simulink model "testRam"  (R2015a)
settings: Solver=ode45  StartTime=0.0  StopTime=10.0  RelTol=1e-3
InitFcn:
  | %% DSPBuilder Start
  | alt_dspbuilder_update_model(bdroot)
  | %% DSPBuilder End
libraries: allblocks_alteradspbuilder2 x35
settings Model: Creator=ASUS  LastModifiedBy=ASUS

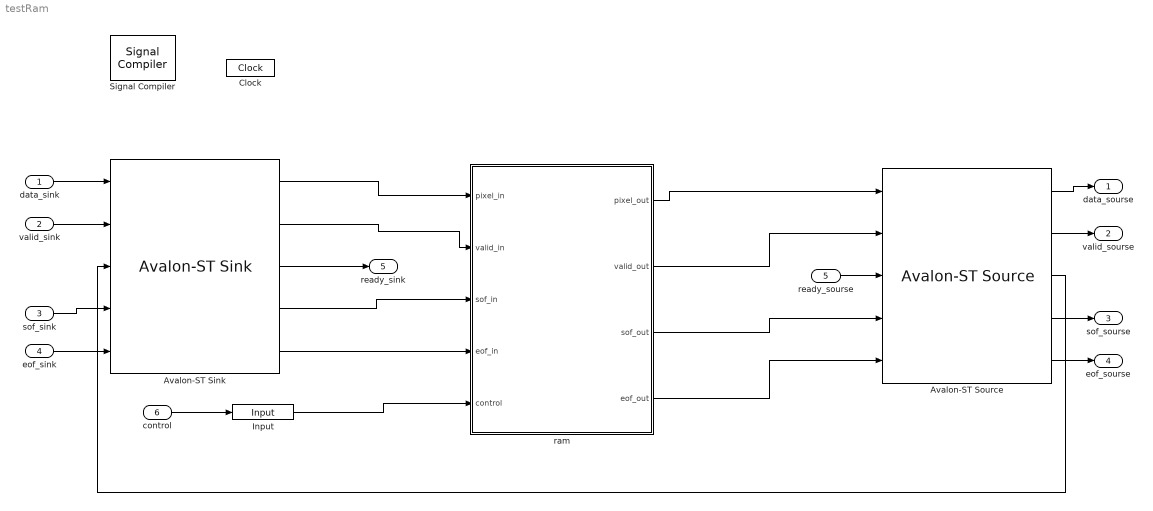
== system testRam ==
  data_sink : Inport
  valid_sink : Inport  Port=2
  sof_sink : Inport  Port=3
  eof_sink : Inport  Port=4
  ready_sourse : Inport  Port=5
  control : Inport  Port=6
  Avalon-ST Sink : allblocks_alteradspbuilder2/Avalon-ST Sink  iofile=C:\Users\ASUS\Desktop\sift_fpga\Octave_2\tb_testRam\testRam_Avalon-ST+Sink_data.salt,C:\Users\ASUS\Desktop\sift_fpga\Octave_2\tb_testRam\testRam_Avalon-ST+Sink_valid.salt,C:\Users\ASUS\Desktop\sift_fpga\Octave_2\tb_testRam\testRam_Avalon-ST+Sink_ready.capture,C:\Users\ASUS\Desktop\sift_fpga\Octave_2\tb_testRam\testRam_Avalon-ST+Sink_startofpacket.salt,C:\Users\ASUS\Desktop\sift_fpga\Octave_2\tb_testRam\testRam_Avalon-ST+Sink_endofpacket.salt,  SpecifyClock=off  BusType=Unsigned Integer  bwl=24  bwr=0  symbolWidth=8  symbolsPerBeat=3  numOfChannels=0  numOfErrorDescriptors=0  endOfPacket=on  startOfPacket=on  empty=off  readyLatency=1  externalType=Inferred  PORTTYPE=Output
  Avalon-ST Source : allblocks_alteradspbuilder2/Avalon-ST Source  iofile=C:\Users\ASUS\Desktop\sift_fpga\Octave_2\tb_testRam\testRam_Avalon-ST+Source_data.capture,C:\Users\ASUS\Desktop\sift_fpga\Octave_2\tb_testRam\testRam_Avalon-ST+Source_valid.capture,C:\Users\ASUS\Desktop\sift_fpga\Octave_2\tb_testRam\testRam_Avalon-ST+Source_ready.salt,C:\Users\ASUS\Desktop\sift_fpga\Octave_2\tb_testRam\testRam_Avalon-ST+Source_startofpacket.capture,C:\Users\ASUS\Desktop\sift_fpga\Octave_2\tb_testRam\testRam_Avalon-ST+Source_endofpacket.capture,  SpecifyClock=off  BusType=Unsigned Integer  bwl=24  bwr=0  symbolWidth=8  symbolsPerBeat=3  numOfChannels=0  numOfErrorDescriptors=0  endOfPacket=on  startOfPacket=on  empty=off  readyLatency=1  externalType=Inferred  PORTTYPE=Input
  Clock : allblocks_alteradspbuilder2/Clock  ClockPeriod=10/1.5  ClockPeriodUnit=ns  SampleTime=1  ResetLatency=0  ResetRegisterCascadeDepth=0  SimulationStartCycle=5  PhaseOffset=0  Reset=aclr  ResetType=Active Low  Export=off
  Input : allblocks_alteradspbuilder2/Input  iofile=C:\Users\ASUS\Desktop\sift_fpga\Octave_2\tb_testRam\testRam_Input.salt  BusType=Unsigned Integer  bwl=18  bwr=0  SpecifyClock=off  PORTTYPE=Input  externalType=Inferred  allowFloatingPointOverride=on  logOutputs=off
  Signal Compiler : allblocks_alteradspbuilder2/Signal Compiler  DeviceFamily=Cyclone IV GX  DeviceName=AUTO  DisableEarlyHDLGeneration=off  EnableSignalTap=off  SignalTapDepth=128  UseBoardBlock=off  StpUseDefaultClock=on  StpClock=Clock  ExportDir=C:\altera\16.0\quartus\dsp_builder  MAX10_ProgrammingMode=Internal Flash (SDM) Single Boot
  ram : Subsystem
  data_sourse : Outport
  valid_sourse : Outport  Port=2
  sof_sourse : Outport  Port=3
  eof_sourse : Outport  Port=4
  ready_sink : Outport  Port=5
  wires:
  ram/1(pixel_out) -> Avalon-ST Source/1
  Avalon-ST Sink/1 -> ram/1(pixel_in)
  Avalon-ST Sink/2 -> ram/2(valid_in)
  ram/2(valid_out) -> Avalon-ST Source/2
  ram/3(sof_out) -> Avalon-ST Source/4
  ram/4(eof_out) -> Avalon-ST Source/5
  Avalon-ST Sink/5 -> ram/4(eof_in)
  Avalon-ST Sink/4 -> ram/3(sof_in)
  Avalon-ST Source/3 -> Avalon-ST Sink/3
  Avalon-ST Source/1 -> data_sourse/1
  Avalon-ST Source/2 -> valid_sourse/1
  Avalon-ST Source/4 -> sof_sourse/1
  Avalon-ST Source/5 -> eof_sourse/1
  data_sink/1 -> Avalon-ST Sink/1
  valid_sink/1 -> Avalon-ST Sink/2
  sof_sink/1 -> Avalon-ST Sink/4
  eof_sink/1 -> Avalon-ST Sink/5
  ready_sourse/1 -> Avalon-ST Source/3
  Avalon-ST Sink/3 -> ready_sink/1
  control/1 -> Input/1
  Input/1 -> ram/5(control)

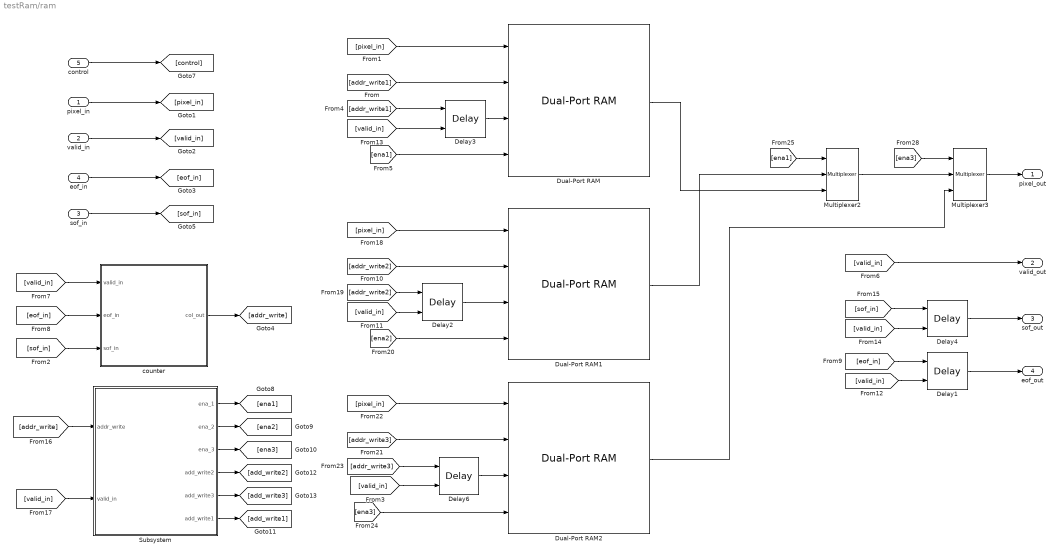
== system testRam/ram ==
  pixel_in : Inport
  valid_in : Inport  Port=2
  sof_in : Inport  Port=3
  eof_in : Inport  Port=4
  control : Inport  Port=5
  Delay1 : allblocks_alteradspbuilder2/Delay  pipeline=5  pipeline_display=5  ClockPhase=1  use_ena=on  use_sclr=off  allowFloatingPointOverride=on  logOutputs=off  logFile=C:\Users\ASUS\Desktop\sift_fpga\Octave_2\tb_testRam\testRam_ram_Delay1.fixedpointlog  use_init=off  reset_value=1
  Delay2 : allblocks_alteradspbuilder2/Delay  pipeline=1  pipeline_display=1  ClockPhase=1  use_ena=on  use_sclr=off  allowFloatingPointOverride=on  logOutputs=off  logFile=C:\Users\ASUS\Desktop\sift_fpga\Octave_2\tb_testRam\testRam_ram_Delay2.fixedpointlog  use_init=off  reset_value=1
  Delay3 : allblocks_alteradspbuilder2/Delay  pipeline=1  pipeline_display=1  ClockPhase=1  use_ena=on  use_sclr=off  allowFloatingPointOverride=on  logOutputs=off  logFile=C:\Users\ASUS\Desktop\sift_fpga\Octave_2\tb_testRam\testRam_ram_Delay3.fixedpointlog  use_init=off  reset_value=1
  Delay4 : allblocks_alteradspbuilder2/Delay  pipeline=5  pipeline_display=5  ClockPhase=1  use_ena=on  use_sclr=off  allowFloatingPointOverride=on  logOutputs=off  logFile=C:\Users\ASUS\Desktop\sift_fpga\Octave_2\tb_testRam\testRam_ram_Delay4.fixedpointlog  use_init=off  reset_value=1
  Delay6 : allblocks_alteradspbuilder2/Delay  pipeline=1  pipeline_display=1  ClockPhase=1  use_ena=on  use_sclr=off  allowFloatingPointOverride=on  logOutputs=off  logFile=C:\Users\ASUS\Desktop\sift_fpga\Octave_2\tb_testRam\testRam_ram_Delay6.fixedpointlog  use_init=off  reset_value=1
  Dual-Port RAM : allblocks_alteradspbuilder2/Dual-Port RAM  numwords=10000  BusType=Unsigned Integer  bwl=24  bwr=0  memory_type=M10K  ram_type=DualRAM  dont_care=off  initialization=Blank  init_file=input.hex  init_array=[0:1:15]  register_outputs=on  use_ena=off  ClockPhase=1  allowFloatingPointOverride=on  logOutputs=off  logFile=C:\Users\ASUS\Desktop\sift_fpga\Octave_2\tb_testRam\testRam_ram_Dual-Port+RAM.fixedpointlog  pipeline_display=2
  Dual-Port RAM1 : allblocks_alteradspbuilder2/Dual-Port RAM  numwords=10000  BusType=Unsigned Integer  bwl=24  bwr=0  memory_type=M10K  ram_type=DualRAM  dont_care=off  initialization=Blank  init_file=input.hex  init_array=[0:1:15]  register_outputs=on  use_ena=off  ClockPhase=1  allowFloatingPointOverride=on  logOutputs=off  logFile=C:\Users\ASUS\Desktop\sift_fpga\Octave_2\tb_testRam\testRam_ram_Dual-Port+RAM1.fixedpointlog  pipeline_display=2
  Dual-Port RAM2 : allblocks_alteradspbuilder2/Dual-Port RAM  numwords=10000  BusType=Unsigned Integer  bwl=24  bwr=0  memory_type=M10K  ram_type=DualRAM  dont_care=off  initialization=Blank  init_file=input.hex  init_array=[0:1:15]  register_outputs=on  use_ena=off  ClockPhase=1  allowFloatingPointOverride=on  logOutputs=off  logFile=C:\Users\ASUS\Desktop\sift_fpga\Octave_2\tb_testRam\testRam_ram_Dual-Port+RAM2.fixedpointlog  pipeline_display=2
  Multiplexer2 : allblocks_alteradspbuilder2/Multiplexer  numInputs=2  pipeline=0  oneHot=off  pipeline_display=0  use_ena=off  use_aclr=off  allowFloatingPointOverride=on  logOutputs=off  logFile=C:\Users\ASUS\Desktop\sift_fpga\Octave_2\tb_testRam\testRam_ram_Multiplexer2.fixedpointlog
  Multiplexer3 : allblocks_alteradspbuilder2/Multiplexer  numInputs=2  pipeline=0  oneHot=off  pipeline_display=0  use_ena=off  use_aclr=off  allowFloatingPointOverride=on  logOutputs=off  logFile=C:\Users\ASUS\Desktop\sift_fpga\Octave_2\tb_testRam\testRam_ram_Multiplexer3.fixedpointlog
  Subsystem : Subsystem
  counter : Subsystem
  pixel_out : Outport
  valid_out : Outport  Port=2
  sof_out : Outport  Port=3
  eof_out : Outport  Port=4
  wires:
  pixel_in/1 -> [pixel_in]
  [pixel_in] -> Dual-Port RAM/1
  [valid_in] -> Delay1/2
  valid_in/1 -> [valid_in]
  eof_in/1 -> [eof_in]
  sof_in/1 -> [sof_in]
  [addr_write1] -> Dual-Port RAM/2
  [valid_in] -> valid_out/1
  [eof_in] -> Delay1/1
  [addr_write1] -> Delay3/1
  [sof_in] -> Delay4/1
  [valid_in] -> Delay4/2
  control/1 -> [control]
  [eof_in] -> counter/2(eof_in)
  [valid_in] -> counter/1(valid_in)
  counter/1(col_out) -> [addr_write]
  Dual-Port RAM/1 -> Multiplexer2/3
  [addr_write] -> Subsystem/1(addr_write)
  [valid_in] -> Subsystem/2(valid_in)
  Subsystem/1(ena_1) -> [ena1]
  Subsystem/2(ena_2) -> [ena2]
  Subsystem/3(ena_3) -> [ena3]
  [ena1] -> Dual-Port RAM/4
  Subsystem/4(add_write2) -> [add_write2]
  Subsystem/5(add_write3) -> [add_write3]
  Subsystem/6(add_write1) -> [add_write1]
  [pixel_in] -> Dual-Port RAM1/1
  [addr_write2] -> Dual-Port RAM1/2
  [addr_write2] -> Delay2/1
  Dual-Port RAM1/1 -> Multiplexer2/2
  [ena2] -> Dual-Port RAM1/4
  [pixel_in] -> Dual-Port RAM2/1
  [addr_write3] -> Dual-Port RAM2/2
  [addr_write3] -> Delay6/1
  [ena3] -> Dual-Port RAM2/4
  [ena1] -> Multiplexer2/1
  Multiplexer2/1 -> Multiplexer3/2
  Dual-Port RAM2/1 -> Multiplexer3/3
  [ena3] -> Multiplexer3/1
  Multiplexer3/1 -> pixel_out/1
  [sof_in] -> counter/3(sof_in)
  Delay1/1 -> eof_out/1
  Delay4/1 -> sof_out/1
  Delay2/1 -> Dual-Port RAM1/3
  Delay3/1 -> Dual-Port RAM/3
  Delay6/1 -> Dual-Port RAM2/3
  [valid_in] -> Delay6/2
  [valid_in] -> Delay2/2
  [valid_in] -> Delay3/2

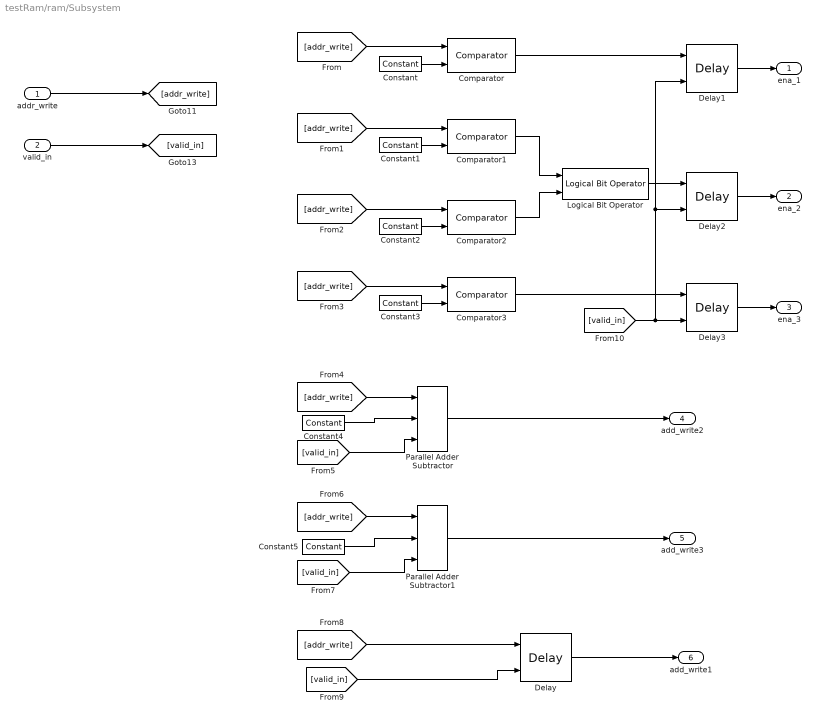
== system testRam/ram/Subsystem ==
  addr_write : Inport
  valid_in : Inport  Port=2
  Comparator : allblocks_alteradspbuilder2/Comparator  direction=a < b  pipeline_display=0  allowFloatingPointOverride=on  logOutputs=off  logFile=C:\Users\ASUS\Desktop\sift_fpga\Octave_2\tb_testRam\testRam_ram_Subsystem_Comparator.fixedpointlog
  Comparator1 : allblocks_alteradspbuilder2/Comparator  direction=a >= b  pipeline_display=0  allowFloatingPointOverride=on  logOutputs=off  logFile=C:\Users\ASUS\Desktop\sift_fpga\Octave_2\tb_testRam\testRam_ram_Subsystem_Comparator1.fixedpointlog
  Comparator2 : allblocks_alteradspbuilder2/Comparator  direction=a < b  pipeline_display=0  allowFloatingPointOverride=on  logOutputs=off  logFile=C:\Users\ASUS\Desktop\sift_fpga\Octave_2\tb_testRam\testRam_ram_Subsystem_Comparator2.fixedpointlog
  Comparator3 : allblocks_alteradspbuilder2/Comparator  direction=a >= b  pipeline_display=0  allowFloatingPointOverride=on  logOutputs=off  logFile=C:\Users\ASUS\Desktop\sift_fpga\Octave_2\tb_testRam\testRam_ram_Subsystem_Comparator3.fixedpointlog
  Constant : allblocks_alteradspbuilder2/Constant  mask_cst=144000  BusType=Signed Integer  bwl=20  bwr=0  roundMode=Truncate  satMode=Wrap  SpecifyClock=off  allowFloatingPointOverride=on  logOutputs=off  logFile=C:\Users\ASUS\Desktop\sift_fpga\Octave_2\tb_testRam\testRam_ram_Subsystem_Constant.fixedpointlog
  Constant1 : allblocks_alteradspbuilder2/Constant  mask_cst=144000  BusType=Signed Integer  bwl=20  bwr=0  roundMode=Truncate  satMode=Wrap  SpecifyClock=off  allowFloatingPointOverride=on  logOutputs=off  logFile=C:\Users\ASUS\Desktop\sift_fpga\Octave_2\tb_testRam\testRam_ram_Subsystem_Constant1.fixedpointlog
  Constant2 : allblocks_alteradspbuilder2/Constant  mask_cst=144000*2  BusType=Signed Integer  bwl=20  bwr=0  roundMode=Truncate  satMode=Wrap  SpecifyClock=off  allowFloatingPointOverride=on  logOutputs=off  logFile=C:\Users\ASUS\Desktop\sift_fpga\Octave_2\tb_testRam\testRam_ram_Subsystem_Constant2.fixedpointlog
  Constant3 : allblocks_alteradspbuilder2/Constant  mask_cst=144000*2  BusType=Signed Integer  bwl=20  bwr=0  roundMode=Truncate  satMode=Wrap  SpecifyClock=off  allowFloatingPointOverride=on  logOutputs=off  logFile=C:\Users\ASUS\Desktop\sift_fpga\Octave_2\tb_testRam\testRam_ram_Subsystem_Constant3.fixedpointlog
  Constant4 : allblocks_alteradspbuilder2/Constant  mask_cst=144000  BusType=Signed Integer  bwl=20  bwr=0  roundMode=Truncate  satMode=Wrap  SpecifyClock=off  allowFloatingPointOverride=on  logOutputs=off  logFile=C:\Users\ASUS\Desktop\sift_fpga\Octave_2\tb_testRam\testRam_ram_Subsystem_Constant4.fixedpointlog
  Constant5 : allblocks_alteradspbuilder2/Constant  mask_cst=144000*2  BusType=Signed Integer  bwl=20  bwr=0  roundMode=Truncate  satMode=Wrap  SpecifyClock=off  allowFloatingPointOverride=on  logOutputs=off  logFile=C:\Users\ASUS\Desktop\sift_fpga\Octave_2\tb_testRam\testRam_ram_Subsystem_Constant5.fixedpointlog
  Delay : allblocks_alteradspbuilder2/Delay  pipeline=1  pipeline_display=1  ClockPhase=1  use_ena=on  use_sclr=off  allowFloatingPointOverride=on  logOutputs=off  logFile=C:\Users\ASUS\Desktop\sift_fpga\Octave_2\tb_testRam\testRam_ram_Subsystem_Delay.fixedpointlog  use_init=off  reset_value=1
  Delay1 : allblocks_alteradspbuilder2/Delay  pipeline=1  pipeline_display=1  ClockPhase=1  use_ena=on  use_sclr=off  allowFloatingPointOverride=on  logOutputs=off  logFile=C:\Users\ASUS\Desktop\sift_fpga\Octave_2\tb_testRam\testRam_ram_Subsystem_Delay1.fixedpointlog  use_init=off  reset_value=1
  Delay2 : allblocks_alteradspbuilder2/Delay  pipeline=1  pipeline_display=1  ClockPhase=1  use_ena=on  use_sclr=off  allowFloatingPointOverride=on  logOutputs=off  logFile=C:\Users\ASUS\Desktop\sift_fpga\Octave_2\tb_testRam\testRam_ram_Subsystem_Delay2.fixedpointlog  use_init=off  reset_value=1
  Delay3 : allblocks_alteradspbuilder2/Delay  pipeline=1  pipeline_display=1  ClockPhase=1  use_ena=on  use_sclr=off  allowFloatingPointOverride=on  logOutputs=off  logFile=C:\Users\ASUS\Desktop\sift_fpga\Octave_2\tb_testRam\testRam_ram_Subsystem_Delay3.fixedpointlog  use_init=off  reset_value=1
  Logical Bit Operator : allblocks_alteradspbuilder2/Logical Bit Operator  LogicalOperator=AND  user_inputs=2  pipeline_display=0
  Parallel Adder Subtractor : allblocks_alteradspbuilder2/Parallel Adder Subtractor  number_of_inputs=2  direction=+-  use_pipeline=on  pipeline_display=1  phase_selection=1  use_ena=on  use_aclr=off  allowFloatingPointOverride=on  logOutputs=off  logFile=C:\Users\ASUS\Desktop\sift_fpga\Octave_2\tb_testRam\testRam_ram_Subsystem_Parallel+Adder+Subtractor.fixedpointlog
  Parallel Adder Subtractor1 : allblocks_alteradspbuilder2/Parallel Adder Subtractor  number_of_inputs=2  direction=+-  use_pipeline=on  pipeline_display=1  phase_selection=1  use_ena=on  use_aclr=off  allowFloatingPointOverride=on  logOutputs=off  logFile=C:\Users\ASUS\Desktop\sift_fpga\Octave_2\tb_testRam\testRam_ram_Subsystem_Parallel+Adder+Subtractor1.fixedpointlog
  ena_1 : Outport
  ena_2 : Outport  Port=2
  ena_3 : Outport  Port=3
  add_write2 : Outport  Port=4
  add_write3 : Outport  Port=5
  add_write1 : Outport  Port=6
  wires:
  addr_write/1 -> [addr_write]
  valid_in/1 -> [valid_in]
  [addr_write] -> Comparator/1
  Constant/1 -> Comparator/2
  Comparator/1 -> Delay1/1
  [addr_write] -> Comparator1/1
  Constant1/1 -> Comparator1/2
  [addr_write] -> Comparator2/1
  Constant2/1 -> Comparator2/2
  Comparator1/1 -> Logical Bit Operator/1
  Comparator2/1 -> Logical Bit Operator/2
  Logical Bit Operator/1 -> Delay2/1
  [addr_write] -> Comparator3/1
  Constant3/1 -> Comparator3/2
  Comparator3/1 -> Delay3/1
  [addr_write] -> Parallel Adder Subtractor/1
  [valid_in] -> Parallel Adder Subtractor/3
  Constant4/1 -> Parallel Adder Subtractor/2
  Parallel Adder Subtractor/1 -> add_write2/1
  [addr_write] -> Parallel Adder Subtractor1/1
  [valid_in] -> Parallel Adder Subtractor1/3
  Constant5/1 -> Parallel Adder Subtractor1/2
  Parallel Adder Subtractor1/1 -> add_write3/1
  [addr_write] -> Delay/1
  Delay/1 -> add_write1/1
  [valid_in] -> Delay/2
  Delay1/1 -> ena_1/1
  Delay2/1 -> ena_2/1
  Delay3/1 -> ena_3/1
  [valid_in] -> Delay1/2, Delay2/2, Delay3/2

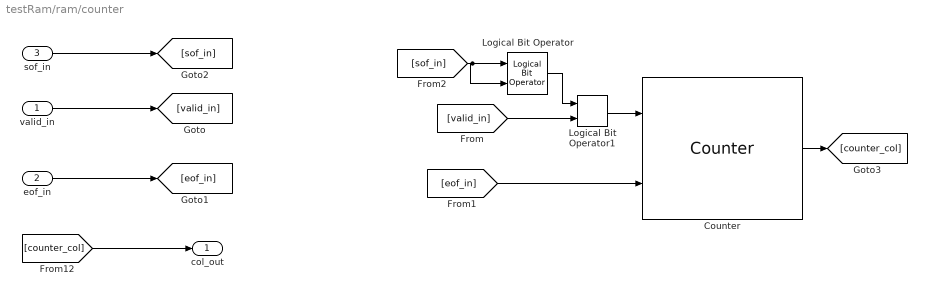
== system testRam/ram/counter ==
  valid_in : Inport
  eof_in : Inport  Port=2
  sof_in : Inport  Port=3
  Counter : allblocks_alteradspbuilder2/Counter  BusType=Unsigned Integer  bwl=19  bwr=0  use_modulo=on  modulo=480*640  SpecifyClock=off  direction=Increment  use_sload=off  use_sset=off  svalue=1  use_clk_ena=off  use_ena=on  use_sclr=on  pipeline_display=1
  Logical Bit Operator : allblocks_alteradspbuilder2/Logical Bit Operator  LogicalOperator=NAND  user_inputs=2  pipeline_display=0
  Logical Bit Operator1 : allblocks_alteradspbuilder2/Logical Bit Operator  LogicalOperator=AND  user_inputs=2  pipeline_display=0
  col_out : Outport
  wires:
  eof_in/1 -> [eof_in]
  valid_in/1 -> [valid_in]
  Counter/1 -> [counter_col]
  [counter_col] -> col_out/1
  [eof_in] -> Counter/2
  [sof_in] -> Logical Bit Operator/2, Logical Bit Operator/1
  [valid_in] -> Logical Bit Operator1/2
  Logical Bit Operator/1 -> Logical Bit Operator1/1
  Logical Bit Operator1/1 -> Counter/1
  sof_in/1 -> [sof_in]
